simulink model "cart_pole"  (R2017a)
settings: Solver=VariableStepAuto  StartTime=0.0  StopTime=20  RelTol=1e-3
values from neighbouring files (symbols this model uses):
  b = 0.05    [No1.mat]    (also in simTest.m)
  be = 0.5    [No1.mat]
  f = 0    [No1.mat]
  g = 9.80665    [No1.mat]    (also in simTest.m)
  K = [1 0]    [No1.mat]    (also in simTest.m = [1;0])
  l = 1    [No1.mat]    (also in animation.m; simTest.m)
  m = 0.5    [No1.mat]    (also in simTest.m)
  M = 1    [No1.mat]    (also in simTest.m)
settings Model: Creator=Sorawit Inprom  LastModifiedBy=Sorawit Inprom

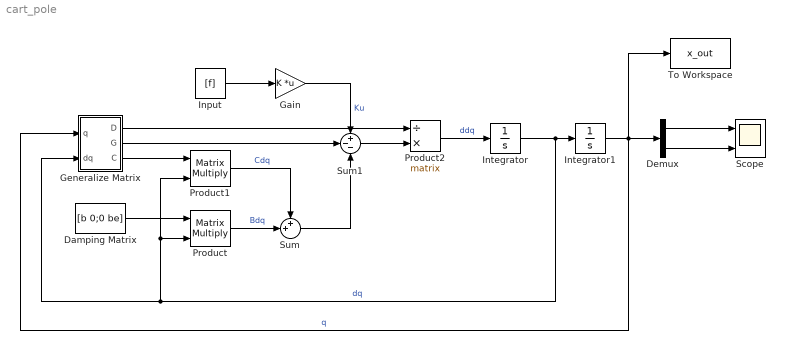
== system cart_pole ==
  Damping Matrix : Constant  Value=[b 0;0 be]
  Demux : Demux  Outputs=2
  Gain : Gain  Gain=K  Multiplication=Matrix(K*u)
  Generalize Matrix : Subsystem
  Input : Constant  Value=[f]
  Integrator : Integrator  InitialCondition=[0;0]
  Integrator1 : Integrator  InitialCondition=[0;pi/4]
  Product : Product  Multiplication=Matrix(*)
  Product1 : Product  Multiplication=Matrix(*)
  Product2 : Product  Inputs=/*  Multiplication=Matrix(*)
  Scope : Scope  NumInputPorts=2
  Sum : Sum  Inputs=++|
  Sum1 : Sum  Inputs=+--
  To Workspace : ToWorkspace  VariableName=x_out  SaveFormat=Timeseries  SampleTime=-1
  wires:
  Product2/1 -> Integrator/1  "ddq"
  Integrator/1 -> Integrator1/1, Generalize Matrix/2(dq), Product1/2, Product/2  "dq"
  Input/1 -> Gain/1
  Damping Matrix/1 -> Product/1
  Sum1/1 -> Product2/2
  Generalize Matrix/1(D) -> Product2/1
  Integrator1/1 -> Demux/1, Generalize Matrix/1(q), To Workspace/1  "q"
  Generalize Matrix/3(C) -> Product1/1
  Product/1 -> Sum/2  "Bdq"
  Product1/1 -> Sum/1  "Cdq"
  Gain/1 -> Sum1/1  "Ku"
  Generalize Matrix/2(G) -> Sum1/2
  Sum/1 -> Sum1/3
  Demux/1 -> Scope/1
  Demux/2 -> Scope/2

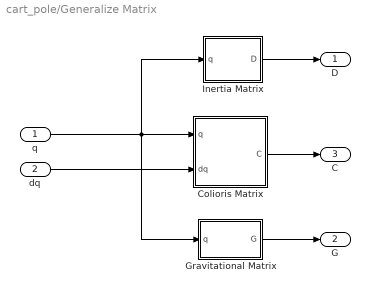
== system cart_pole/Generalize Matrix ==
  q : Inport
  dq : Inport  Port=2
  Colioris Matrix : Subsystem
  Gravitational Matrix : Subsystem
  Inertia Matrix : Subsystem
  D : Outport
  G : Outport  Port=2
  C : Outport  Port=3
  wires:
  Gravitational Matrix/1(G) -> G/1
  Colioris Matrix/1(C) -> C/1
  Inertia Matrix/1(D) -> D/1
  dq/1 -> Colioris Matrix/2(dq)
  q/1 -> Gravitational Matrix/1(q), Inertia Matrix/1(q), Colioris Matrix/1(q)

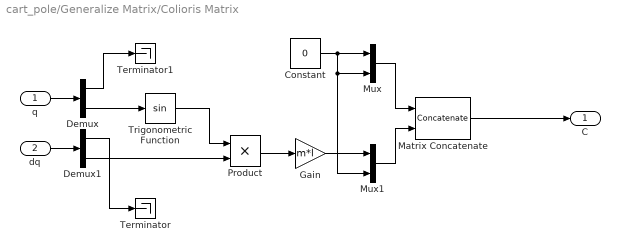
== system cart_pole/Generalize Matrix/Colioris Matrix ==
  q : Inport
  dq : Inport  Port=2
  Constant : Constant  Value=0
  Demux : Demux  Outputs=2
  Demux1 : Demux  Outputs=2
  Gain : Gain  Gain=m*l
  Matrix Concatenate : Concatenate  Mode=Multidimensional array  ConcatenateDimension=2
  Mux : Mux  Inputs=2
  Mux1 : Mux  Inputs=2
  Product : Product
  Terminator : Terminator
  Terminator1 : Terminator
  Trigonometric Function : Trigonometry
  C : Outport
  wires:
  Mux1/1 -> Matrix Concatenate/2
  Demux/2 -> Trigonometric Function/1
  q/1 -> Demux/1
  dq/1 -> Demux1/1
  Product/1 -> Gain/1
  Gain/1 -> Mux1/1
  Mux/1 -> Matrix Concatenate/1
  Matrix Concatenate/1 -> C/1
  Demux1/2 -> Product/2
  Constant/1 -> Mux1/2, Mux/2, Mux/1
  Trigonometric Function/1 -> Product/1
  Demux/1 -> Terminator1/1
  Demux1/1 -> Terminator/1

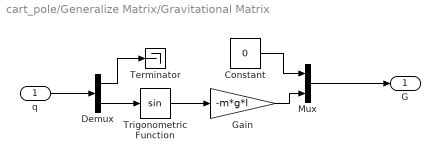
== system cart_pole/Generalize Matrix/Gravitational Matrix ==
  q : Inport
  Constant : Constant  Value=0
  Demux : Demux  Outputs=2
  Gain : Gain  Gain=-m*g*l
  Mux : Mux  Inputs=2
  Terminator : Terminator
  Trigonometric Function : Trigonometry
  G : Outport
  wires:
  Trigonometric Function/1 -> Gain/1
  Demux/1 -> Terminator/1
  Constant/1 -> Mux/1
  Gain/1 -> Mux/2
  q/1 -> Demux/1
  Mux/1 -> G/1
  Demux/2 -> Trigonometric Function/1

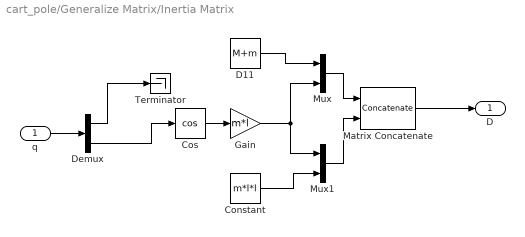
== system cart_pole/Generalize Matrix/Inertia Matrix ==
  q : Inport
  Constant : Constant  Value=m*l*l
  Cos : Trigonometry  Operator=cos
  D11 : Constant  Value=M+m
  Demux : Demux  Outputs=2
  Gain : Gain  Gain=m*l
  Matrix Concatenate : Concatenate  Mode=Multidimensional array  ConcatenateDimension=2
  Mux : Mux  Inputs=2
  Mux1 : Mux  Inputs=2
  Terminator : Terminator
  D : Outport
  wires:
  Gain/1 -> Mux1/1, Mux/2
  D11/1 -> Mux/1
  Cos/1 -> Gain/1
  Matrix Concatenate/1 -> D/1
  Mux/1 -> Matrix Concatenate/1
  Mux1/1 -> Matrix Concatenate/2
  Constant/1 -> Mux1/2
  q/1 -> Demux/1
  Demux/1 -> Terminator/1
  Demux/2 -> Cos/1
